simulink model "ParallelBuckLQILoadChange"  (R2018b)
settings: Solver=ode23tb  StartTime=0.0  StopTime=1  RelTol=1e-3
undefined symbols (not defined in the file): C, K, Ki, L1, L2, R, rL1, rL2, Vi1, Vi2
libraries: powerlib x18, powerlib_meascontrol x2
settings Model: Creator=Charles-Spencer  LastModifiedBy=Charles-Spencer

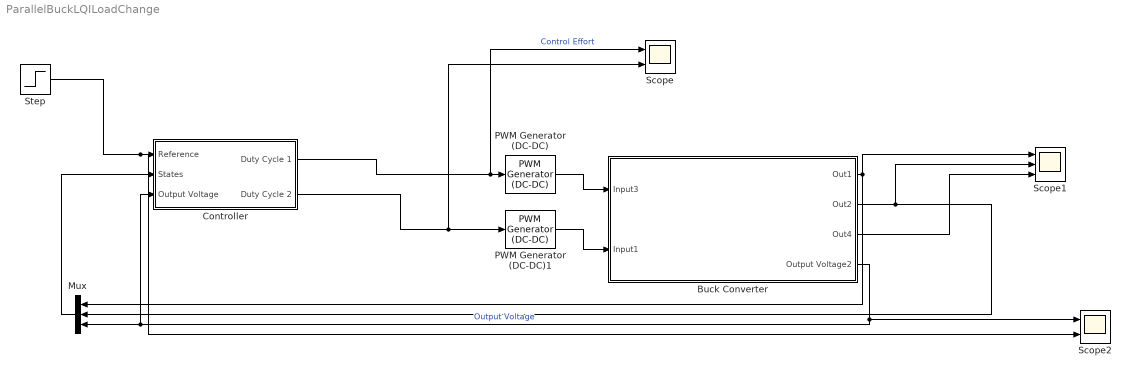
== system ParallelBuckLQILoadChange ==
  Buck Converter : Subsystem
  Controller : Subsystem
  Mux : Mux  Inputs=3
  PWM Generator (DC-DC) : powerlib_meascontrol/Pulse & Signal Generators/PWM Generator (DC-DC)  Fsw=fsw  Ts=0
  PWM Generator (DC-DC)1 : powerlib_meascontrol/Pulse & Signal Generators/PWM Generator (DC-DC)  Fsw=fsw  Ts=0
  Scope : Scope  NumInputPorts=2
  Scope1 : Scope  NumInputPorts=3
  Scope2 : Scope  NumInputPorts=2
  Step : Step  Before=48  After=48  SampleTime=0
  wires:
  PWM Generator (DC-DC)1/1 -> Buck Converter/2(Input1)
  PWM Generator (DC-DC)/1 -> Buck Converter/1(Input3)
  Buck Converter/1(Out1) -> Scope1/1, Mux/1
  Buck Converter/2(Out2) -> Scope1/2, Mux/2
  Buck Converter/4(Output Voltage2) -> Controller/3(Output Voltage), Mux/3, Scope2/1  "Output Voltage"
  Controller/1(Duty Cycle 1) -> Scope/1, PWM Generator (DC-DC)/1  "Control Effort"
  Step/1 -> Scope2/2, Controller/1(Reference)
  Controller/2(Duty Cycle 2) -> Scope/2, PWM Generator (DC-DC)1/1
  Mux/1 -> Controller/2(States)
  Buck Converter/3(Out4) -> Scope1/3

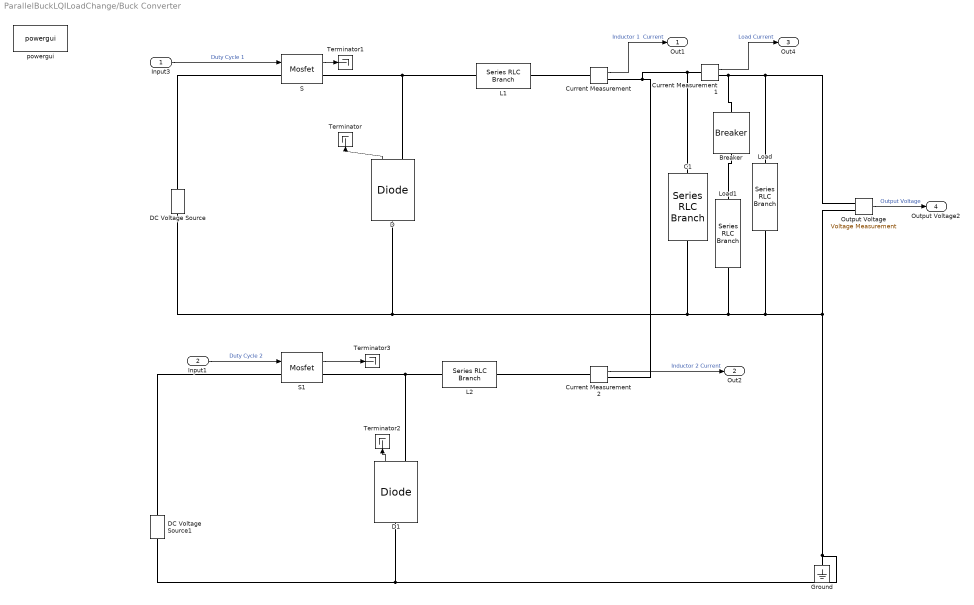
== system ParallelBuckLQILoadChange/Buck Converter ==
  Input3 : Inport
  Input1 : Inport  Port=2
  Breaker : powerlib/Elements/Breaker  InitialState=0  SwitchingTimes=0.5  External=off  BreakerResistance=0.01  SnubberResistance=1e6  SnubberCapacitance=inf  Measurements=None  MoreParameters=on  NoBreakLoop=off
      settings: SourceProductName=Simscape Power Systems
  C1 : powerlib/Elements/Series RLC Branch  LConnTagsString=__new0  RConnTagsString=__new0  BranchType=C  Resistance=1  Inductance=1e-3  SetiL0=off  InitialCurrent=0  Capacitance=C  Setx0=off  InitialVoltage=0  Measurements=None
      settings: SourceProductName=Simscape Electrical
  Current Measurement : powerlib/Measurements/Current Measurement  PhasorSimulation=off  OutputType=Complex  PSBequivalent=0
      settings: SourceProductName=Simscape Electrical
  Current Measurement1 : powerlib/Measurements/Current Measurement  PhasorSimulation=off  OutputType=Complex  PSBequivalent=0
      settings: SourceProductName=Simscape Electrical
  Current Measurement2 : powerlib/Measurements/Current Measurement  PhasorSimulation=off  OutputType=Complex  PSBequivalent=0
      settings: SourceProductName=Simscape Electrical
  D : powerlib/Power Electronics/Diode  Ron=0.0001  Lon=0  Vf=0  IC=0  UseSnubber=off  Rs=5000  Cs=250e-9  Measurements=on
      settings: SourceProductName=Simscape Electrical
  D1 : powerlib/Power Electronics/Diode  Ron=0.0001  Lon=0  Vf=0  IC=0  UseSnubber=off  Rs=5000  Cs=250e-9  Measurements=on
      settings: SourceProductName=Simscape Electrical
  DC Voltage Source : powerlib/Electrical Sources/DC Voltage Source  Amplitude=Vi1  Measurements=None
  DC Voltage Source1 : powerlib/Electrical Sources/DC Voltage Source  Amplitude=Vi2  Measurements=None
  Ground : powerlib/Elements/Ground  LConnTagsString=a
  L1 : powerlib/Elements/Series RLC Branch  LConnTagsString=__new0  RConnTagsString=__new0  BranchType=RL  Resistance=rL1  Inductance=L1  SetiL0=off  InitialCurrent=0  Capacitance=1e-6  Setx0=off  InitialVoltage=0  Measurements=None
      settings: SourceProductName=Simscape Electrical
  L2 : powerlib/Elements/Series RLC Branch  LConnTagsString=__new0  RConnTagsString=__new0  BranchType=RL  Resistance=rL2  Inductance=L2  SetiL0=off  InitialCurrent=0  Capacitance=1e-6  Setx0=off  InitialVoltage=0  Measurements=None
      settings: SourceProductName=Simscape Electrical
  Load : powerlib/Elements/Series RLC Branch  LConnTagsString=__new0  RConnTagsString=__new0  BranchType=R  Resistance=R  Inductance=1e-3  SetiL0=off  InitialCurrent=0  Capacitance=1e-6  Setx0=off  InitialVoltage=0  Measurements=None
      settings: SourceProductName=Simscape Electrical
  Load1 : powerlib/Elements/Series RLC Branch  LConnTagsString=__new0  RConnTagsString=__new0  BranchType=R  Resistance=2*R  Inductance=1e-3  SetiL0=off  InitialCurrent=0  Capacitance=1e-6  Setx0=off  InitialVoltage=0  Measurements=None
      settings: SourceProductName=Simscape Electrical
  Output Voltage : powerlib/Measurements/Voltage Measurement  PhasorSimulation=off  OutputType=Complex  PSBequivalent=0
      settings: SourceProductName=Simscape Electrical
  S : powerlib/Power Electronics/Mosfet  Ron=0.001  Lon=0  Rd=0.0001  Vfd=0  IC=0  Rs=1e5  Cs=inf  Measurements=on
      settings: SourceProductName=Simscape Electrical
  S1 : powerlib/Power Electronics/Mosfet  Ron=0.001  Lon=0  Rd=0.0001  Vfd=0  IC=0  Rs=1e5  Cs=inf  Measurements=on
      settings: SourceProductName=Simscape Electrical
  Terminator{,1..3} (4 alike) : Terminator
  powergui : powerlib/powergui  Priority=1  SimulationMode=Continuous  SampleTime=50e-7  frequency=60  Iterations=50  frequencyindice=0  Pbase=100e6  ErrMax=1e-4  UnitsV=kV  UnitsW=MW  buscounter=0  FunctionMessages=off  echomessages=off  EnableUseOfTLC=off  CurrentSourceSwitches=off  DisableSnubberDevices=off  DisableRonSwitches=off  DisableVfSwitches=off  DisplayEquations=off  SolverType=Tustin/Backward Euler (TBE)  Interpol=off  ExternalGateDelay=off  methode=off  Ts=100  x0status=blocks  SPID=on  SwTol=0  HookPort=off  RestoreLinks=warning  ResistiveCurrentMeasurement=off  Frange=[0:2:500]  Ylog=off  Xlog=on  ShowGrid=off  save=off  variable=ZData  structure=0  ZoomFFT=off  StartTime=0.0  cycles=1  DisplayStyle=1  fundamental=60  FreqAxis=off  MaxFrequency=1000  frequencyindicesteady=1  RmsSteady=1  display=off
  Out1 : Outport
  Out2 : Outport  Port=2
  Out4 : Outport  Port=3
  Output Voltage2 : Outport  Port=4
  wires:
  Current Measurement1/1 -> Out4/1  "Load Current"
  Output Voltage/1 -> Output Voltage2/1  "Output Voltage"
  Current Measurement/1 -> Out1/1  "Inductor 1  Current"
  Input3/1 -> S/1  "Duty Cycle 1"
  D/1 -> Terminator/1
  S/1 -> Terminator1/1
  D1/1 -> Terminator2/1
  Input1/1 -> S1/1  "Duty Cycle 2"
  Current Measurement2/1 -> Out2/1  "Inductor 2 Current"
  S1/1 -> Terminator3/1
  connections:
  Current Measurement1/RConn1 -- Output Voltage/LConn1 -- Load/LConn1 -- Breaker/RConn1
  Current Measurement2/RConn1 -- C1/LConn1 -- Current Measurement1/LConn1 -- Current Measurement/RConn1
  Load1/RConn1 -- DC Voltage Source/LConn1 -- D/LConn1 -- C1/RConn1 -- Load/RConn1 -- Output Voltage/LConn2 -- DC Voltage Source1/LConn1 -- D1/LConn1 -- Ground/LConn1
  L1/LConn1 -- D/RConn1 -- S/RConn1
  L1/RConn1 -- Current Measurement/LConn1
  DC Voltage Source/RConn1 -- S/LConn1
  D1/RConn1 -- S1/RConn1 -- L2/LConn1
  L2/RConn1 -- Current Measurement2/LConn1
  S1/LConn1 -- DC Voltage Source1/RConn1
  Breaker/LConn1 -- Load1/LConn1

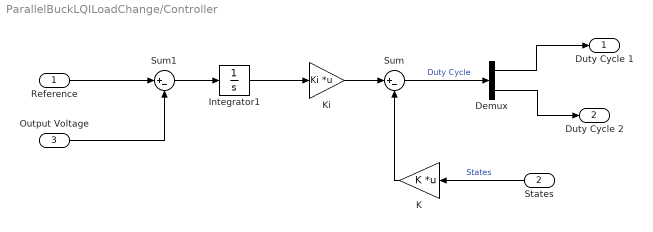
== system ParallelBuckLQILoadChange/Controller ==
  Reference : Inport
  States : Inport  Port=2
  Output Voltage : Inport  Port=3
  Demux : Demux  Outputs=2
  Integrator1 : Integrator
  K : Gain  Gain=K  Multiplication=Matrix(K*u)
  Ki : Gain  Gain=Ki  Multiplication=Matrix(K*u)
  Sum : Sum  Inputs=|+-
  Sum1 : Sum  Inputs=|+-
  Duty Cycle 1 : Outport
  Duty Cycle 2 : Outport  Port=2
  wires:
  Integrator1/1 -> Ki/1
  Reference/1 -> Sum1/1
  States/1 -> K/1  "States"
  Sum1/1 -> Integrator1/1
  Output Voltage/1 -> Sum1/2
  Ki/1 -> Sum/1
  K/1 -> Sum/2
  Sum/1 -> Demux/1  "Duty Cycle"
  Demux/1 -> Duty Cycle 1/1
  Demux/2 -> Duty Cycle 2/1
